simulink model "bio_matfunc_omega_mat"  (R2017b)
settings: Solver=VariableStepAuto  StartTime=0.0  StopTime=10.0  RelTol=1e-3
settings Model: Creator=ktrinh  LastModifiedBy=ktrinh

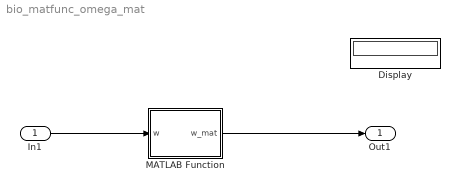
== system bio_matfunc_omega_mat ==
  In1 : Inport  OutDataTypeStr=double  PortDimensions=3
  Display : Display
  MATLAB Function : MATLAB Function  TreatAsAtomicUnit=on
  Out1 : Outport
  wires:
  In1/1 -> MATLAB Function/1(w)
  MATLAB Function/1(w_mat) -> Out1/1

== matlab function bio_matfunc_omega_mat/MATLAB Function ==
  data: w input; w_mat output
function w_mat = omega_mat(w)

w_mat = 0.5*[0  w(3)  -w(2)  w(1);
             -w(3)  0  w(1)   w(2);
             w(2)  -w(1)  0  w(3);
             -w(1) -w(2) -w(3) 0];
